simulink model "Clutchless_P2_Parallel_ETE"  (R2017b)
settings: Solver=FixedStepAuto  StartTime=0.0  StopTime=length(Speed)  FixedStep=0.01  MaxStep=0.01  RelTol=1e-3  EnableMultiTasking=on
PostLoadFcn:
  | , if any(exist('dsrtsu_mdlpostloadfcn', 'file') == [2, 3, 6]), try dsrtsu_mdlpostloadfcn('Execute', bdroot); catch fprintf('Error in PostLoadFcn (dsrtsu_mdlpostloadfcn) for model "%s":\n %s\n', bdroot, lasterr); end, end,
undefined symbols (not defined in the file): ABSEnable, Actuators, air, APP1_OOR, APP2_OOR, APP_Mismatch, Brk_Flt, cal, ClutchEngag, Clutchless_HSC_ETE, CS_On_Control, Driver, eng, Engine, EngOverTemp, ENGTRQ_MSMCH_Degraded_CP, ENGTRQ_MSMCH_ErrCritical_CP, ENGTRQ_MSMCH_LimpHome_CP, EngTrqMismatch, env, ess, ESSOverTemp, gb, KeyPos_Flt, KeyPosition, lib_Actuators, lib_Clutchless_HSC_ETE, lib_Driver, lib_EMachine_2017a, lib_Sensors_2017a, LossCAN, Machine, max_vehicle_rad_air_flow, MCUOverTemp, mot, MotDirMismatch, MotOverTemp, MotTrqMismatch, mph2ms, PRNDL_Flt, RegenBrkDisable, RegenFault, Sensors, ShiftLeverPosition, Speed, SW_CS_ON, SW_Engine_ON, t_amb, time, tloop
libraries: simulink x97, Pneumatic_lib x11, nesl_utility x9, EC2_libraries x7, powerlib_meascontrol x2, CalculationGallon x1, lib_Chassis x1, lib_DCDC x1, lib_Differential x1, lib_HVESS x1, fl_lib x1, lib_OBC x1
(part 8 of 9)

== system Clutchless_P2_Parallel_ETE/Clutchless_HSC_ETE/HSC/Camaro Fault Detection/Signal Diagnostic/Driver Signal Diagnostic/BrakeFailureDetection ==
  BPP : Inport
  VehSpeed : Inport  Port=2
  Trigger : TriggerPort  VariantControl=Variant  PortDimensions=1
  Chart : Stateflow chart  Commented=on  TreatAsAtomicUnit=on
  Compare To Constant : simulink/Logic and Bit Operations/Compare To Constant  relop=>  const=0  OutDataTypeStr=boolean
  Compare To Constant1 : simulink/Logic and Bit Operations/Compare To Constant  relop=>  const=0.5  OutDataTypeStr=boolean
  Detect Change : simulink/Logic and Bit Operations/Detect Change  vinit=0  InputProcessing=Inherited  OutDataTypeStr=boolean
  Detect Increase : simulink/Logic and Bit Operations/Detect Increase  vinit=0.0  InputProcessing=Inherited  OutDataTypeStr=boolean
  Logical Operator : Logic  Operator=NOT  AllPortsSameDT=off  OutDataTypeStr=boolean
  Logical Operator1 : Logic  AllPortsSameDT=off  OutDataTypeStr=boolean
  Logical Operator2 : Logic  Operator=OR  AllPortsSameDT=off  OutDataTypeStr=boolean
  Logical Operator3 : Logic  AllPortsSameDT=off  OutDataTypeStr=boolean
  Unit Delay : UnitDelay  SampleTime=-1
  Unit Delay1 : UnitDelay  SampleTime=-1
  DecelFail : Outport
  wires:
  VehSpeed/1 -> Unit Delay1/1, Detect Change/1, Detect Increase/1
  Detect Change/1 -> Logical Operator/1
  Compare To Constant/1 -> Logical Operator1/1
  Compare To Constant1/1 -> Logical Operator1/2
  BPP/1 -> Unit Delay/1
  Logical Operator1/1 -> Logical Operator3/1
  Detect Increase/1 -> Logical Operator2/1  "Increase"
  Logical Operator/1 -> Logical Operator2/2  "Unchange"
  Unit Delay/1 -> Compare To Constant/1
  Unit Delay1/1 -> Compare To Constant1/1
  Logical Operator2/1 -> Logical Operator3/2
  Logical Operator3/1 -> DecelFail/1

== system Clutchless_P2_Parallel_ETE/Clutchless_HSC_ETE/HSC/Camaro Fault Detection/Signal Diagnostic/Driver Signal Diagnostic/Latch ==
  In1 : Inport
  In2 : Inport  Port=2
  Memory : Memory
  NOT : Logic  Operator=NOT  OutDataTypeStr=boolean
  OR : Logic  OutDataTypeStr=boolean
  OR1 : Logic  Operator=OR  OutDataTypeStr=boolean
  Drv_APP_Agree : Outport
  wires:
  In1/1 -> OR1/1
  OR/1 -> OR1/2
  OR1/1 -> Drv_APP_Agree/1, Memory/1
  NOT/1 -> OR/1
  Memory/1 -> OR/2
  In2/1 -> NOT/1

== system Clutchless_P2_Parallel_ETE/Clutchless_HSC_ETE/HSC/Camaro Fault Detection/Signal Diagnostic/Driver Signal Diagnostic/Latch1 ==
  In1 : Inport
  In2 : Inport  Port=2
  Memory : Memory
  NOT : Logic  Operator=NOT  OutDataTypeStr=boolean
  OR : Logic  OutDataTypeStr=boolean
  OR1 : Logic  Operator=OR  OutDataTypeStr=boolean
  Out1 : Outport
  wires:
  In2/1 -> NOT/1
  Memory/1 -> OR/2
  NOT/1 -> OR/1
  OR1/1 -> Memory/1, Out1/1
  OR/1 -> OR1/2
  In1/1 -> OR1/1

== system Clutchless_P2_Parallel_ETE/Clutchless_HSC_ETE/HSC/Camaro Fault Detection/Signal Diagnostic/ESS Signal Diagnostic/Contactors status check ==
  note: Note: Contactors don't close when commanded
  In1 : Inport
  In2 : Inport  Port=2
  In3 : Inport  Port=3
  " " : simulink/Logic and Bit Operations/Compare To Constant  relop=>  const=0.5  OutDataTypeStr=boolean
  Abs : Abs
  Logical Operator : Logic  Operator=OR  AllPortsSameDT=off  OutDataTypeStr=boolean
  Sum : Sum  Inputs=+-
  Out1 : Outport
  wires:
  " "/1 -> Logical Operator/1  "BMS_contactorsFailed_SigValid"
  In3/1 -> Logical Operator/2
  In2/1 -> Sum/2
  Abs/1 -> " "/1
  Sum/1 -> Abs/1
  Logical Operator/1 -> Out1/1  "BMS_contactorsFailed_Detected"
  In1/1 -> Sum/1

== system Clutchless_P2_Parallel_ETE/Clutchless_HSC_ETE/HSC/Camaro Fault Detection/Signal Diagnostic/ESS Signal Diagnostic/ESS SOC Validity Check ==
  In1 : Inport
  Constant1 : Constant
  essSOCValidity_Check : Subsystem
  essSOC_0_1Range : Stateflow chart  TreatAsAtomicUnit=on
  Out1 : Outport
  Out2 : Outport  Port=2
  wires:
  essSOCValidity_Check/1(Out1) -> Out1/1  "BMS_essSOC_0_1_SigValid"
  In1/1 -> essSOC_0_1Range/2(signalValue)
  Constant1/1 -> essSOC_0_1Range/1(clearFaults)
  essSOC_0_1Range/1(essSOCRange) -> Out2/1, essSOCValidity_Check/1(In1)

== system Clutchless_P2_Parallel_ETE/Clutchless_HSC_ETE/HSC/Camaro Fault Detection/Signal Diagnostic/ESS Signal Diagnostic/ESS Temp Validity Check ==
  In1 : Inport
  Constant : Constant
  essTsignalRange : Stateflow chart  TreatAsAtomicUnit=on
  essTsignalValidity_Check : Subsystem
  Out1 : Outport
  Out2 : Outport  Port=2
  wires:
  Constant/1 -> essTsignalRange/1(clearFaults)
  essTsignalValidity_Check/1(Out1) -> Out1/1  "BMS_essTemp_[degC]_SigValid"
  essTsignalRange/1(essTempRange) -> Out2/1, essTsignalValidity_Check/1(In1)  "essTempRange[0_4]"
  In1/1 -> essTsignalRange/2(signalValue)

== system Clutchless_P2_Parallel_ETE/Clutchless_HSC_ETE/HSC/Camaro Fault Detection/Signal Diagnostic/ESS Signal Diagnostic/Max charging voltage fault detect ==
  note: Note: When the ESS receives the energy from grid or regenerative braking,
      | the charging voltage to the inverter can not be bigger than 419V, otherwise the MCU will set to fault
  In1 : Inport
  " " : simulink/Logic and Bit Operations/Compare To Constant  relop=>  const=419  OutDataTypeStr=boolean
  Abs : Abs
  Compare To Zero : simulink/Logic and Bit Operations/Compare To Zero  relop=<  OutDataTypeStr=boolean
  Logical Operator : Logic  AllPortsSameDT=off  OutDataTypeStr=boolean
  Out1 : Outport
  wires:
  Compare To Zero/1 -> Logical Operator/2
  In1/1 -> Abs/1, Compare To Zero/1
  " "/1 -> Logical Operator/1
  Logical Operator/1 -> Out1/1
  Abs/1 -> " "/1

== system Clutchless_P2_Parallel_ETE/Clutchless_HSC_ETE/HSC/Camaro Fault Detection/Signal Diagnostic/ESS Signal Diagnostic/Rolling Alive Counter Detection ==
  In1 : Inport
  Chart : Stateflow chart  TreatAsAtomicUnit=on
  Constant : Constant  Value=0.01
  Constant1 : Constant  Value=0.01
  Detect Change : simulink/Logic and Bit Operations/Detect Change  vinit=1  InputProcessing=Inherited  OutDataTypeStr=boolean
  Out1 : Outport
  wires:
  Constant/1 -> Chart/2(CycleTime)
  Chart/1(flag) -> Out1/1
  Detect Change/1 -> Chart/1(PulseDetect)
  In1/1 -> Detect Change/1
  Constant1/1 -> Chart/3(tloop)

== system Clutchless_P2_Parallel_ETE/Clutchless_HSC_ETE/HSC/Camaro Fault Detection/Signal Diagnostic/ESS Signal Diagnostic/Validity Check ==
  In1 : Inport
  " Normal Operation" : simulink/Logic and Bit Operations/Compare To Constant  relop===  const=1  OutDataTypeStr=boolean
  Below Normal Operation : simulink/Logic and Bit Operations/Compare To Constant  relop===  const=0  OutDataTypeStr=boolean
  Logical Operator : Logic  Operator=OR  AllPortsSameDT=off  OutDataTypeStr=boolean
  Out1 : Outport
  wires:
  Logical Operator/1 -> Out1/1  "BMSgdf_SigValid"
  " Normal Operation"/1 -> Logical Operator/2
  Below Normal Operation/1 -> Logical Operator/1
  In1/1 -> " Normal Operation"/1, Below Normal Operation/1

== system Clutchless_P2_Parallel_ETE/Clutchless_HSC_ETE/HSC/Camaro Fault Detection/Signal Diagnostic/Engine Signal Diagnostic/EngTempValidity_Check ==
  In1 : Inport
  Above Normal Operation : simulink/Logic and Bit Operations/Compare To Constant  relop===  const=3  OutDataTypeStr=boolean
  Logical Operator1 : Logic  Operator=NOT  AllPortsSameDT=off  OutDataTypeStr=boolean
  Out1 : Outport
  wires:
  In1/1 -> Above Normal Operation/1
  Above Normal Operation/1 -> Logical Operator1/1
  Logical Operator1/1 -> Out1/1

== system Clutchless_P2_Parallel_ETE/Clutchless_HSC_ETE/HSC/Camaro Fault Detection/Signal Diagnostic/Engine Signal Diagnostic/Rolling Alive Counter Detection1 ==
  In1 : Inport
  Chart : Stateflow chart  TreatAsAtomicUnit=on
  Constant : Constant  Value=0.01
  Detect Change : simulink/Logic and Bit Operations/Detect Change  vinit=1  InputProcessing=Inherited  OutDataTypeStr=boolean
  Out1 : Outport
  wires:
  In1/1 -> Detect Change/1
  Detect Change/1 -> Chart/1(PulseDetect)
  Chart/1(flag) -> Out1/1
  Constant/1 -> Chart/2(CycleTime)

== system Clutchless_P2_Parallel_ETE/Clutchless_HSC_ETE/HSC/Camaro Fault Detection/Signal Diagnostic/Transmission Signal Diagnostic/Rolling Alive Counter Detection ==
  In1 : Inport
  Chart : Stateflow chart  TreatAsAtomicUnit=on
  Constant : Constant  Value=0.01
  Detect Change : simulink/Logic and Bit Operations/Detect Change  vinit=1  InputProcessing=Inherited  OutDataTypeStr=boolean
  Out1 : Outport
  wires:
  In1/1 -> Detect Change/1
  Detect Change/1 -> Chart/1(PulseDetect)
  Chart/1(flag) -> Out1/1
  Constant/1 -> Chart/2(CycleTime)

== system Clutchless_P2_Parallel_ETE/Clutchless_HSC_ETE/HSC/Camaro Fault Detection/Signal Diagnostic/Transmission Signal Diagnostic/Vehicle Direction Fault Detection ==
  LvrPosTrnsShft : Inport
  Speed : Inport  Port=2
  Compare To Constant : simulink/Logic and Bit Operations/Compare To Constant  relop===  const=4  OutDataTypeStr=boolean
  Compare To Constant1 : simulink/Logic and Bit Operations/Compare To Constant  relop=<  const=0  OutDataTypeStr=boolean
  Compare To Constant2 : simulink/Logic and Bit Operations/Compare To Constant  relop===  const=2  OutDataTypeStr=boolean
  Compare To Constant3 : simulink/Logic and Bit Operations/Compare To Constant  relop=>  const=0  OutDataTypeStr=boolean
  Logical Operator : Logic  AllPortsSameDT=off  OutDataTypeStr=boolean
  Logical Operator1 : Logic  AllPortsSameDT=off  OutDataTypeStr=boolean
  Logical Operator2 : Logic  Operator=OR  AllPortsSameDT=off  OutDataTypeStr=boolean
  Out1 : Outport
  wires:
  LvrPosTrnsShft/1 -> Compare To Constant2/1, Compare To Constant/1
  Speed/1 -> Compare To Constant3/1, Compare To Constant1/1
  Compare To Constant1/1 -> Logical Operator/2
  Compare To Constant/1 -> Logical Operator/1
  Compare To Constant2/1 -> Logical Operator1/1
  Compare To Constant3/1 -> Logical Operator1/2
  Logical Operator1/1 -> Logical Operator2/1
  Logical Operator/1 -> Logical Operator2/2
  Logical Operator2/1 -> Out1/1

== system Clutchless_P2_Parallel_ETE/Clutchless_HSC_ETE/HSC/Driver_Requests/APP_BPP to DrvIntndAxlTrq2/Post Driver Intnded Axle Torque/Brake Command ==
  APP : Inport
  BPP : Inport  Port=2
  VehicleSpeed : Inport  Port=3
  1-D Lookup Table : Lookup_n-D  NumberOfTableDimensions=1  BreakpointsForDimension1=cal.Regen.BrakeAxleTrq.idx1_BrkPdlPos  Table=cal.Regen.BrakeAxleTrq.map  InternalRulePriority=Speed  RndMeth=Simplest  InputSameDT=on
  Compare To Constant : simulink/Logic and Bit Operations/Compare To Constant  relop=>=  const=cal.Regen.EnableSpeed  OutDataTypeStr=boolean
  Compare To Constant4 : simulink/Logic and Bit Operations/Compare To Constant  relop=<=  const=cal.Regen.EnableAPP  OutDataTypeStr=boolean
  Compare To Constant5 : simulink/Logic and Bit Operations/Compare To Constant  relop=>=  const=cal.Regen.DisableAPP  OutDataTypeStr=boolean
  Constant5 : Constant  Value=0
  Latch : Subsystem
  RegenCal : Gain  Gain=1.3
  Switch : Switch  Criteria=u2 > Threshold  Threshold=1
  Terminator : Terminator
  BrkAxlTrq : Outport
  wires:
  RegenCal/1 -> Switch/1
  Latch/1(Out1) -> Terminator/1
  Compare To Constant4/1 -> Latch/1(Input)
  Compare To Constant5/1 -> Latch/2(Reset)
  Constant5/1 -> Switch/3
  Compare To Constant/1 -> Switch/2
  BPP/1 -> 1-D Lookup Table/1
  APP/1 -> Compare To Constant4/1, Compare To Constant5/1
  Switch/1 -> BrkAxlTrq/1
  1-D Lookup Table/1 -> RegenCal/1
  VehicleSpeed/1 -> Compare To Constant/1

== system Clutchless_P2_Parallel_ETE/Clutchless_HSC_ETE/HSC/Driver_Requests/APP_BPP to DrvIntndAxlTrq2/Post Driver Intnded Axle Torque/Driver Intended Axle Torque ==
  note: //*mode==1 (CD Mode)
      | mode==2 (CS Mode - Engine Drive)
      | mode==3 (CS Mode-Motor Drive) pass MotTrq
      | mode==4 (Sports Mode) pass Mot Trq+Eng Trq
      | mode==5 (Engine Charging mode)
      | mode==66 (Engine Only mode)*//
  note: In Engine Only mode, ETAS is only as a gateway to broadcast CAN messages
  APP : Inport
  Mode : Inport  Port=2
  TransGearRatio : Inport  Port=3
  Compare To Constant1 : simulink/Logic and Bit Operations/Compare To Constant  relop===  const=2  OutDataTypeStr=boolean
  Compare To Constant2 : simulink/Logic and Bit Operations/Compare To Constant  relop===  const=4  OutDataTypeStr=boolean
  Compare To Constant3 : simulink/Logic and Bit Operations/Compare To Constant  relop===  const=5  OutDataTypeStr=boolean
  Compare To Constant4 : simulink/Logic and Bit Operations/Compare To Constant  relop===  const=1  OutDataTypeStr=boolean
  Compare To Constant5 : simulink/Logic and Bit Operations/Compare To Constant  relop===  const=3  OutDataTypeStr=boolean
  Compare To Constant6 : simulink/Logic and Bit Operations/Compare To Constant  relop===  const=66  OutDataTypeStr=boolean
  Constant : Constant  Value=eng.plant.trq_max_hot_point  VectorParams1D=off
  Constant1 : Constant  Value=fd.plant.init.ratio
  Constant2 : Constant  Value=mot.plant.init.motor.trq_max.points.trq  VectorParams1D=off
  Constant3 : Constant  Value=mot.plant.init.motor.trq_max.points.trq  VectorParams1D=off
  Constant4 : Constant  Value=eng.plant.trq_max_hot_point  VectorParams1D=off
  Gain1 : Gain  Gain=1/100
  Gain2 : Gain  Gain=1/100
  Gain3 : Gain  Gain=1/100
  Logical Operator : Logic  Operator=OR  Inputs=4  AllPortsSameDT=off  OutDataTypeStr=boolean
  Logical Operator1 : Logic  Operator=OR  AllPortsSameDT=off  OutDataTypeStr=boolean
  Memory : Memory
  Product : Product  RndMeth=Zero
  Product1 : Product  RndMeth=Zero
  Product2 : Product  Inputs=3  RndMeth=Zero
  Product3 : Product  RndMeth=Zero
  Ratio Filter : Subsystem
  Sum1 : Sum
  Switch1 : Switch  Threshold=1
  Switch3 : Switch  Threshold=1
  Out1 : Outport
  wires:
  Compare To Constant5/1 -> Logical Operator/4
  Compare To Constant4/1 -> Logical Operator/3
  Compare To Constant6/1 -> Logical Operator1/2
  Logical Operator1/1 -> Switch1/2
  Gain3/1 -> Product3/1
  Constant4/1 -> Product3/2
  APP/1 -> Gain1/1, Gain3/1, Gain2/1
  Memory/1 -> Compare To Constant5/1, Compare To Constant4/1, Compare To Constant1/1, Compare To Constant6/1, Compare To Constant3/1, Compare To Constant2/1
  Compare To Constant3/1 -> Logical Operator1/1
  Switch1/1 -> Product2/1
  Product3/1 -> Switch1/1, [IntdAxleTrq_eng]
  Logical Operator/1 -> Switch3/2
  Switch3/1 -> Switch1/3  "DrvIntndAxlTrq"
  Constant/1 -> Sum1/2
  Compare To Constant2/1 -> Logical Operator/2
  Sum1/1 -> Product/1
  Compare To Constant1/1 -> Logical Operator/1
  Constant3/1 -> Sum1/1
  Gain1/1 -> Product/2
  Product2/1 -> Out1/1  "DrvIntndAxlTrq"
  TransGearRatio/1 -> Ratio Filter/1(Ratio)
  Product1/1 -> Switch3/3
  Constant1/1 -> Product2/3  "ratio"
  Mode/1 -> Memory/1
  Product/1 -> Switch3/1
  Gain2/1 -> Product1/2
  Ratio Filter/1(Filtered_Ratio) -> Product2/2
  Constant2/1 -> Product1/1

== system Clutchless_P2_Parallel_ETE/Clutchless_HSC_ETE/HSC/Powertrain Manager/HV Manager1/BMS_Manager/Fault Latch ==
  IsoFault : Inport
  Off Delay : powerlib_meascontrol/Logic/On Delay  DelayType=Off delay  delay=3  ic=0  Ts=0
      settings: SourceProductName=Simscape Power Systems
  IsoFaultLatched : Outport
  wires:
  Off Delay/1 -> IsoFaultLatched/1
  IsoFault/1 -> Off Delay/1

== system Clutchless_P2_Parallel_ETE/Clutchless_HSC_ETE/HSC/Powertrain Manager/HV Manager1/BMS_Manager/ISO_Hybrid_01_Req ==
  In1 : Inport
  Bus Creator : BusCreator  Inputs=9
  ISO_Hybrid_01_Req_Data_byte_0 : Constant  Value=3
  ISO_Hybrid_01_Req_Data_byte_1 : Constant  Value=34
  ISO_Hybrid_01_Req_Data_byte_2 : Constant  Value=30
  ISO_Hybrid_01_Req_Data_byte_3 : Constant  Value=25
  ISO_Hybrid_01_Req_Data_byte_{4..7} (4 alike) : Constant  Value=0
  ISO_Hybrid_01_Req_Data_byte_8 : Constant  Value=23
  ISO_Request : DiscretePulseGenerator  PulseType=Time based  Period=0.5  PulseWidth=50  SampleTime=-1
  Switch{,1..8} (9 alike) : Switch  Criteria=u2 > Threshold
  Out1 : Outport
  wires:
  ISO_Request/1 -> Switch/2  "<ISO_Hybrid_01_Req_Data_byte_3>"
  ISO_Hybrid_01_Req_Data_byte_7/1 -> Switch8/1
  ISO_Hybrid_01_Req_Data_byte_6/1 -> Switch7/1
  ISO_Hybrid_01_Req_Data_byte_5/1 -> Switch6/1
  ISO_Hybrid_01_Req_Data_byte_4/1 -> Switch5/1
  Switch/1 -> Switch4/1  "ISO_Hybrid_01_Req_Data_byte_3"
  ISO_Hybrid_01_Req_Data_byte_2/1 -> Switch3/1
  ISO_Hybrid_01_Req_Data_byte_1/1 -> Switch2/1
  In1/1 -> Switch1/2, Switch1/3, Switch2/3, Switch3/2, Switch4/2, Switch5/2, Switch6/2, Switch8/3, Bus Creator/9, Switch8/2, Switch7/3, Switch7/2, Switch6/3, Switch5/3, Switch4/3, Switch3/3, Switch2/2
  ISO_Hybrid_01_Req_Data_byte_0/1 -> Switch1/1
  Switch4/1 -> Bus Creator/4  "ISO_Hybrid_01_Req_Data_byte_3"
  Switch8/1 -> Bus Creator/8  "ISO_Hybrid_01_Req_Data_byte_7"
  Switch2/1 -> Bus Creator/2  "ISO_Hybrid_01_Req_Data_byte_1"
  Switch7/1 -> Bus Creator/7  "ISO_Hybrid_01_Req_Data_byte_6"
  Switch1/1 -> Bus Creator/1  "ISO_Hybrid_01_Req_Data_byte_0"
  ISO_Hybrid_01_Req_Data_byte_3/1 -> Switch/1
  Switch3/1 -> Bus Creator/3  "ISO_Hybrid_01_Req_Data_byte_2"
  Switch5/1 -> Bus Creator/5  "ISO_Hybrid_01_Req_Data_byte_4"
  ISO_Hybrid_01_Req_Data_byte_8/1 -> Switch/3
  Switch6/1 -> Bus Creator/6  "ISO_Hybrid_01_Req_Data_byte_5"
  Bus Creator/1 -> Out1/1  "ISO_Hybrid_01_Req"

== system Clutchless_P2_Parallel_ETE/Clutchless_HSC_ETE/HSC/Powertrain Manager/HV Manager1/BMS_Manager/Isolation Fault Calculation ==
  note: This block  allows to know which HV main
      | is having issues. HV POS 25, HV NEG 23.
  Sensors1 : Inport
  Bus Selector5 : BusSelector  OutputSignals=from_CAN.fromEBCAN.from_BMSAntrieb.ISO_Hybrid_01_Resp_Data.ISO_Hybrid_01_Resp_Data_byte_3,from_CAN.fromEBCAN.from_BMSAntrieb.ISO_Hybrid_01_Resp_Data.ISO_Hybrid_01_Resp_Data_byte_4,from_CAN.fromEBCAN.from_BMSAntrieb.ISO_Hybrid_01_Resp_Data.ISO_Hybrid_01_Resp_Data_byte_5
  Compare To Constant : simulink/Logic and Bit Operations/Compare To Constant  relop===  const=23  OutDataTypeStr=boolean
  Compare To Constant1 : simulink/Logic and Bit Operations/Compare To Constant  relop===  const=25  OutDataTypeStr=boolean
  HVnegativeISO : Constant  Value=0
  HVpositiveISO : Constant
  Logical Operator : Logic  Operator=OR  AllPortsSameDT=off  OutDataTypeStr=boolean
  POS or NEG HV MAIN : Switch  Criteria=u2 > Threshold  Threshold=24
  Resistance_Measurement : Subsystem
  Terminator8 : Terminator
  IsoFault : Outport
  wires:
  Logical Operator/1 -> Resistance_Measurement/Enable
  Compare To Constant/1 -> Logical Operator/2
  Compare To Constant1/1 -> Logical Operator/1
  HVnegativeISO/1 -> POS or NEG HV MAIN/3
  Bus Selector5/1 -> Compare To Constant/1, Compare To Constant1/1, POS or NEG HV MAIN/2  "<ISO_Hybrid_01_Resp_Data_byte_3>"
  HVpositiveISO/1 -> POS or NEG HV MAIN/1
  Sensors1/1 -> Bus Selector5/1
  Bus Selector5/3 -> Resistance_Measurement/2(In2)  "<ISO_Hybrid_01_Resp_Data_byte_5>"
  Bus Selector5/2 -> Resistance_Measurement/1(In1)  "<ISO_Hybrid_01_Resp_Data_byte_4>"
  POS or NEG HV MAIN/1 -> Terminator8/1
  Resistance_Measurement/1(IsoFault) -> IsoFault/1

== system Clutchless_P2_Parallel_ETE/Clutchless_HSC_ETE/HSC/Powertrain Manager/HV Manager1/DCDC Manager/Contactors status check ==
  note: Note: Contactors don't close when commanded
  In1 : Inport
  " " : simulink/Logic and Bit Operations/Compare To Constant  relop=>  const=5  OutDataTypeStr=boolean
  Abs : Abs
  Bus Selector1 : BusSelector  OutputSignals=from_CAN.fromHV_CAN.from_BMSHybrid.BMS_HYB_02.BMS_IstSpannung,from_CAN.fromHV_CAN.from_BMSHybrid.BMS_Spannung_ZwKr,from_CAN.fromHV_CAN.from_BMSHybrid.BMS_HYB_02.BMS_Fehler_Pilot
  Logical Operator : Logic  Operator=OR  AllPortsSameDT=off  OutDataTypeStr=boolean
  Sum : Sum  Inputs=+-
  Out1 : Outport
  wires:
  Bus Selector1/2 -> Sum/2  "<BMS_Spannung_ZwKr>"
  Bus Selector1/3 -> Logical Operator/2  "<BMS_Fehler_Pilot>"
  In1/1 -> Bus Selector1/1
  " "/1 -> Logical Operator/1  "BMS_contactorsFailed_SigValid"
  Abs/1 -> " "/1
  Sum/1 -> Abs/1
  Logical Operator/1 -> Out1/1  "BMS_contactorsFailed_Detected"
  Bus Selector1/1 -> Sum/1  "<BMS_IstSpannung>"

== system Clutchless_P2_Parallel_ETE/Clutchless_HSC_ETE/HSC/Powertrain Manager/HV Manager1/DCDC Manager/Override_Current ==
  In1 : Inport
  CurrentHVOvrrdSW : Constant  Value=0
  CurrentHVOvrrdVAL : Constant  Value=20
  Switch : Switch  Criteria=u2 > Threshold
  Out1 : Outport
  wires:
  CurrentHVOvrrdVAL/1 -> Switch/1
  CurrentHVOvrrdSW/1 -> Switch/2
  In1/1 -> Switch/3
  Switch/1 -> Out1/1  "DC_mode"

== system Clutchless_P2_Parallel_ETE/Clutchless_HSC_ETE/HSC/Powertrain Manager/HV Manager1/DCDC Manager/Override_CurrentLV ==
  In1 : Inport
  CurrentLVOvrrdSW : Constant  Value=0
  CurrentLVOvrrdVAL : Constant  Value=173
  Switch : Switch  Criteria=u2 > Threshold
  Out1 : Outport
  wires:
  CurrentLVOvrrdVAL/1 -> Switch/1
  CurrentLVOvrrdSW/1 -> Switch/2
  In1/1 -> Switch/3
  Switch/1 -> Out1/1  "DC_mode"

== system Clutchless_P2_Parallel_ETE/Clutchless_HSC_ETE/HSC/Powertrain Manager/HV Manager1/DCDC Manager/Override_Voltage ==
  In1 : Inport
  Switch : Switch  Criteria=u2 > Threshold
  VoltageHVOvrrdSW : Constant  Value=0
  voltageHVOvrrdVal : Constant  Value=0
  Out1 : Outport
  wires:
  Switch/1 -> Out1/1  "DC_mode"
  In1/1 -> Switch/3
  VoltageHVOvrrdSW/1 -> Switch/2
  voltageHVOvrrdVal/1 -> Switch/1

== system Clutchless_P2_Parallel_ETE/Clutchless_HSC_ETE/HSC/Powertrain Manager/HV Manager1/DCDC Manager/Override_VoltageLV ==
  In1 : Inport
  Switch : Switch  Criteria=u2 > Threshold
  VoltageLVOvrrdSW : Constant  Value=0
  VoltageLVOvrrdVAL : Constant  Value=14
  Out1 : Outport
  wires:
  Switch/1 -> Out1/1  "DC_mode"
  In1/1 -> Switch/3
  VoltageLVOvrrdSW/1 -> Switch/2
  VoltageLVOvrrdVAL/1 -> Switch/1

== system Clutchless_P2_Parallel_ETE/Clutchless_HSC_ETE/HSC/Powertrain Manager/HV Manager1/DCDC Manager/Override_mode ==
  In1 : Inport
  DCDCOVrrdSwitch : Constant  Value=0
  DCDCOVrrdVal : Constant  Value=0
  Switch : Switch  Criteria=u2 > Threshold
  Out1 : Outport
  wires:
  DCDCOVrrdVal/1 -> Switch/1
  DCDCOVrrdSwitch/1 -> Switch/2
  In1/1 -> Switch/3
  Switch/1 -> Out1/1  "DC_mode"

== system Clutchless_P2_Parallel_ETE/Clutchless_HSC_ETE/HSC/Powertrain Manager/Torque Distribution/AxlTrq_to_EngTrq/Ratio Filter ==
  Ratio : Inport
  Abs : Abs
  Compare To Zero : simulink/Logic and Bit Operations/Compare To Zero  relop===  OutDataTypeStr=boolean
  Constant : Constant  Value=cal.Time.TrnsOvrllEstTrqRatioSwitch
  Mature_Delay : EC2_libraries/Mature_Delay
  Memory1 : Memory  InitialCondition=1
  Switch1 : Switch  Threshold=1
  Switch2 : Switch  Threshold=1
  Filtered_Ratio : Outport
  wires:
  Switch2/1 -> Memory1/1, Filtered_Ratio/1  "gear_ratio"
  Memory1/1 -> Switch1/3
  Mature_Delay/1 -> Switch1/2
  Constant/1 -> Mature_Delay/2
  Switch1/1 -> Switch2/1
  Abs/1 -> Switch2/3, Switch1/1
  Compare To Zero/1 -> Switch2/2, Mature_Delay/1
  Ratio/1 -> Abs/1, Compare To Zero/1

== system Clutchless_P2_Parallel_ETE/Clutchless_HSC_ETE/HSC/Powertrain Manager/Torque Distribution/AxlTrq_to_MotTrq/AxlTrq_to_MtrTrq2 ==
  note: //From motor axle torque to motor torque//
  In1 : Inport
  Compare To Constant : simulink/Logic and Bit Operations/Compare To Constant  relop===  const=0  OutDataTypeStr=boolean
  Constant1 : Constant  Value=max(gb.plant.init.ratio.map)
  Constant5 : Constant  Value=fd.plant.init.ratio
  Divide : Product  Inputs=*//
  Rate Limiter : RateLimiter  RisingSlewLimit=mcu.plant.init.trq_uprate  FallingSlewLimit=mcu.plant.init.trq_derate
  Ratio Filter : Subsystem
  Switch : Switch  Criteria=u2 > Threshold
  MtrTrqCmd : Outport
  wires:
  Ratio Filter/1(Filtered_Ratio) -> Compare To Constant/1, Switch/3
  Switch/1 -> Divide/3
  Rate Limiter/1 -> MtrTrqCmd/1
  Constant1/1 -> Switch/1
  Compare To Constant/1 -> Switch/2
  [TransRatio] -> Ratio Filter/1(Ratio)
  Divide/1 -> Rate Limiter/1
  Constant5/1 -> Divide/2
  In1/1 -> Divide/1

== system Clutchless_P2_Parallel_ETE/Clutchless_HSC_ETE/HSC/Powertrain Manager/Torque Distribution/AxlTrq_to_MotTrq/electric machine filter ==
  trq : Inport
  Interval Test : simulink/Logic and Bit Operations/Interval Test  IntervalClosedRight=on  uplimit=0.02  IntervalClosedLeft=on  lowlimit=-0.02  OutDataTypeStr=boolean
  Switch : Switch  Threshold=0.5
  electric machine time response : TransferFcn  Denominator=[mot.plant.init.time_response 1]
  filtered : Outport
  wires:
  Switch/1 -> filtered/1
  trq/1 -> Switch/1, electric machine time response/1, Interval Test/1
  Interval Test/1 -> Switch/2
  electric machine time response/1 -> Switch/3

== system Clutchless_P2_Parallel_ETE/Clutchless_HSC_ETE/HSC/Powertrain Manager/Torque Distribution/Supervisory  Control  Logic/VehReady.Eng_Charging_Stat.EngTrqCalc/Multiply by Zero Fix ==
  In1 : Inport
  Compare To Constant : simulink/Logic and Bit Operations/Compare To Constant  relop===  const=0  OutDataTypeStr=boolean
  Constant1 : Constant  Value=max(gb.plant.init.ratio.map)
  Ratio Filter : Subsystem
  Switch : Switch  Criteria=u2 > Threshold
  Out1 : Outport
  wires:
  In1/1 -> Ratio Filter/1(Ratio)
  Constant1/1 -> Switch/1
  Switch/1 -> Out1/1
  Compare To Constant/1 -> Switch/2
  Ratio Filter/1(Filtered_Ratio) -> Compare To Constant/1, Switch/3

== system Clutchless_P2_Parallel_ETE/Camaro Plant Model/E-Machine/IMG Plant/Electric Machine/Thermal1/MotInv_loop/MCUOverTemp Fault ==
  In1 : Inport
  Gain : Gain  Gain=3
  Switch : Switch  Threshold=1
  Out1 : Outport
  wires:
  Switch/1 -> Out1/1
  Gain/1 -> Switch/1
  [MCUOverTemp] -> Switch/2
  In1/1 -> Gain/1, Switch/3

== system Clutchless_P2_Parallel_ETE/Camaro Plant Model/E-Machine/IMG Plant/Electric Machine/Thermal1/MotInv_loop/MotorOverTempFault ==
  In1 : Inport
  Gain : Gain  Gain=2
  Memory : Memory
  Switch1 : Switch  Threshold=1
  Out1 : Outport
  wires:
  Switch1/1 -> Out1/1
  Gain/1 -> Switch1/1
  [MotOverTemp] -> Switch1/2
  In1/1 -> Switch1/3, Memory/1
  Memory/1 -> Gain/1

== system Clutchless_P2_Parallel_ETE/Camaro Plant Model/E-Machine/IMG Plant/Electric Machine/Thermal1/Motor Thermal/Lower Limit ==
  In1 : Inport
  Constant3 : Constant  Value=Lolimit
  MinMax : MinMax  Function=max  Inputs=2
  Out1 : Outport
  wires:
  MinMax/1 -> Out1/1
  Constant3/1 -> MinMax/2
  In1/1 -> MinMax/1

== system Clutchless_P2_Parallel_ETE/Camaro Plant Model/E-Machine/Soft MCU/Torque Calculation1/max torque /Heat index/Divide ==
  note: Take care of
      | division by 0
  numerator : Inport
  denominator : Inport  Port=2
  Fcn : Fcn  Expr=u[1] / ( u[2] + eps*(u[2]==0) )
  Mux : Mux  Inputs=2
  quotient : Outport
  wires:
  denominator/1 -> Mux/2
  Fcn/1 -> quotient/1
  numerator/1 -> Mux/1
  Mux/1 -> Fcn/1

== system Clutchless_P2_Parallel_ETE/Camaro Plant Model/E-Machine/Soft MCU/Torque Calculation2/max torque /Heat index/Divide ==
  note: Take care of
      | division by 0
  numerator : Inport
  denominator : Inport  Port=2
  Fcn : Fcn  Expr=u[1] / ( u[2] + eps*(u[2]==0) )
  Mux : Mux  Inputs=2
  quotient : Outport
  wires:
  denominator/1 -> Mux/2
  Fcn/1 -> quotient/1
  numerator/1 -> Mux/1
  Mux/1 -> Fcn/1

== system Clutchless_P2_Parallel_ETE/Clutchless_HSC_ETE/HSC/Camaro Fault Detection/Signal Diagnostic/ESS Signal Diagnostic/ESS SOC Validity Check/essSOCValidity_Check ==
  In1 : Inport
  Above Normal Operation : simulink/Logic and Bit Operations/Compare To Constant  relop===  const=3  OutDataTypeStr=boolean
  Below Normal Operation : simulink/Logic and Bit Operations/Compare To Constant  relop===  const=0  OutDataTypeStr=boolean
  Logical Operator : Logic  Operator=OR  AllPortsSameDT=off  OutDataTypeStr=boolean
  Logical Operator1 : Logic  Operator=NOT  AllPortsSameDT=off  OutDataTypeStr=boolean
  Out1 : Outport
  wires:
  Logical Operator1/1 -> Out1/1
  Above Normal Operation/1 -> Logical Operator/2
  Below Normal Operation/1 -> Logical Operator/1
  Logical Operator/1 -> Logical Operator1/1
  In1/1 -> Below Normal Operation/1, Above Normal Operation/1

== system Clutchless_P2_Parallel_ETE/Clutchless_HSC_ETE/HSC/Camaro Fault Detection/Signal Diagnostic/ESS Signal Diagnostic/ESS Temp Validity Check/essTsignalValidity_Check ==
  In1 : Inport
  Above Normal Operation : simulink/Logic and Bit Operations/Compare To Constant  relop===  const=4  OutDataTypeStr=boolean
  Below Normal Operation : simulink/Logic and Bit Operations/Compare To Constant  relop===  const=0  OutDataTypeStr=boolean
  Logical Operator : Logic  Operator=OR  AllPortsSameDT=off  OutDataTypeStr=boolean
  Logical Operator1 : Logic  Operator=NOT  AllPortsSameDT=off  OutDataTypeStr=boolean
  Out1 : Outport
  wires:
  In1/1 -> Above Normal Operation/1, Below Normal Operation/1
  Logical Operator/1 -> Logical Operator1/1
  Below Normal Operation/1 -> Logical Operator/1
  Above Normal Operation/1 -> Logical Operator/2
  Logical Operator1/1 -> Out1/1

== system Clutchless_P2_Parallel_ETE/Clutchless_HSC_ETE/HSC/Driver_Requests/APP_BPP to DrvIntndAxlTrq2/Post Driver Intnded Axle Torque/Brake Command/Latch ==
  Input : Inport
  Reset : Inport  Port=2
  Logical Operator1 : Logic  Operator=NOT  AllPortsSameDT=off  OutDataTypeStr=boolean
  Logical Operator2 : Logic  AllPortsSameDT=off  OutDataTypeStr=boolean
  Logical Operator3 : Logic  Operator=OR  AllPortsSameDT=off  OutDataTypeStr=boolean
  Memory1 : Memory
  Out1 : Outport
  wires:
  Input/1 -> Logical Operator3/1
  Logical Operator1/1 -> Logical Operator2/1
  Logical Operator3/1 -> Memory1/1, Out1/1
  Memory1/1 -> Logical Operator2/2
  Reset/1 -> Logical Operator1/1
  Logical Operator2/1 -> Logical Operator3/2

== system Clutchless_P2_Parallel_ETE/Clutchless_HSC_ETE/HSC/Driver_Requests/APP_BPP to DrvIntndAxlTrq2/Post Driver Intnded Axle Torque/Driver Intended Axle Torque/Ratio Filter ==
  Ratio : Inport
  Abs : Abs
  Compare To Zero : simulink/Logic and Bit Operations/Compare To Zero  relop===  OutDataTypeStr=boolean
  Constant : Constant  Value=cal.Time.TrnsOvrllEstTrqRatioSwitch
  Mature_Delay : EC2_libraries/Mature_Delay
  Memory1 : Memory  InitialCondition=1
  Switch1 : Switch  Threshold=1
  Switch2 : Switch  Threshold=1
  Filtered_Ratio : Outport
  wires:
  Switch2/1 -> Memory1/1, Filtered_Ratio/1  "gear_ratio"
  Memory1/1 -> Switch1/3
  Mature_Delay/1 -> Switch1/2
  Constant/1 -> Mature_Delay/2
  Switch1/1 -> Switch2/1
  Abs/1 -> Switch2/3, Switch1/1
  Compare To Zero/1 -> Switch2/2, Mature_Delay/1
  Ratio/1 -> Abs/1, Compare To Zero/1

== system Clutchless_P2_Parallel_ETE/Clutchless_HSC_ETE/HSC/Powertrain Manager/HV Manager1/BMS_Manager/Isolation Fault Calculation/Resistance_Measurement ==
  In1 : Inport
  In2 : Inport  Port=2
  Enable : EnablePort
  Add : Sum
  ISOfault : Constant
  ISOmultiplier : Constant  Value=256
  ISOnofault : Constant  Value=0
  Minimum Allowed Isolation Resistance : Switch  Criteria=u2 > Threshold  Threshold=500000
  Product : Product
  Product1 : Product
  Resistance Adjustment : Constant  Value=1000
  IsoFault : Outport
  wires:
  ISOmultiplier/1 -> Product/2
  In1/1 -> Product/1
  In2/1 -> Add/2
  Product/1 -> Add/1
  Add/1 -> Product1/1
  ISOfault/1 -> Minimum Allowed Isolation Resistance/3
  Product1/1 -> Minimum Allowed Isolation Resistance/2
  Resistance Adjustment/1 -> Product1/2
  ISOnofault/1 -> Minimum Allowed Isolation Resistance/1
  Minimum Allowed Isolation Resistance/1 -> IsoFault/1  "IsoFault"

== system Clutchless_P2_Parallel_ETE/Clutchless_HSC_ETE/HSC/Powertrain Manager/Torque Distribution/AxlTrq_to_MotTrq/AxlTrq_to_MtrTrq2/Ratio Filter ==
  Ratio : Inport
  Abs : Abs
  Compare To Zero : simulink/Logic and Bit Operations/Compare To Zero  relop===  OutDataTypeStr=boolean
  Constant : Constant  Value=cal.Time.TrnsOvrllEstTrqRatioSwitch
  Mature_Delay : EC2_libraries/Mature_Delay
  Memory1 : Memory  InitialCondition=1
  Switch1 : Switch  Threshold=1
  Switch2 : Switch  Threshold=1
  Filtered_Ratio : Outport
  wires:
  Switch2/1 -> Memory1/1, Filtered_Ratio/1  "gear_ratio"
  Memory1/1 -> Switch1/3
  Mature_Delay/1 -> Switch1/2
  Constant/1 -> Mature_Delay/2
  Switch1/1 -> Switch2/1
  Abs/1 -> Switch2/3, Switch1/1
  Compare To Zero/1 -> Switch2/2, Mature_Delay/1
  Ratio/1 -> Abs/1, Compare To Zero/1

== system Clutchless_P2_Parallel_ETE/Clutchless_HSC_ETE/HSC/Powertrain Manager/Torque Distribution/Supervisory  Control  Logic/VehReady.Eng_Charging_Stat.EngTrqCalc/Multiply by Zero Fix/Ratio Filter ==
  Ratio : Inport
  Abs : Abs
  Compare To Zero : simulink/Logic and Bit Operations/Compare To Zero  relop===  OutDataTypeStr=boolean
  Constant : Constant  Value=cal.Time.TrnsOvrllEstTrqRatioSwitch
  Mature_Delay : Subsystem  AncestorBlock=EC2_libraries/Mature_Delay
  Memory1 : Memory  InitialCondition=1  InheritSampleTime=on
  Switch1 : Switch  Threshold=1
  Switch2 : Switch  Threshold=1
  Filtered_Ratio : Outport
  wires:
  Switch2/1 -> Memory1/1, Filtered_Ratio/1  "gear_ratio"
  Memory1/1 -> Switch1/3
  Mature_Delay/1(Out) -> Switch1/2
  Constant/1 -> Mature_Delay/2(MatTime)
  Switch1/1 -> Switch2/1
  Abs/1 -> Switch2/3, Switch1/1
  Compare To Zero/1 -> Switch2/2, Mature_Delay/1(In)
  Ratio/1 -> Abs/1, Compare To Zero/1

== system Clutchless_P2_Parallel_ETE/Clutchless_HSC_ETE/HSC/Powertrain Manager/Torque Distribution/Supervisory  Control  Logic/VehReady.Eng_Charging_Stat.EngTrqCalc/Multiply by Zero Fix/Ratio Filter/Mature_Delay ==
  In : Inport
  MatTime : Inport  Port=2
  Gain : Gain  Gain=-1
  Lower Limit : EC2_libraries/Lower Limit  Lolimit=0.001
  Memory1 : Memory  InheritSampleTime=on
  Relational Operator1 : RelationalOperator  Operator=>  OutDataTypeStr=boolean  RndMeth=Nearest
  StepTm[sec] : Constant  Value=tloop
  Sum : Sum  Inputs=|++
  Switch1 : Switch  Threshold=1
  Out : Outport
  wires:
  In/1 -> Switch1/2
  Gain/1 -> Switch1/3
  Memory1/1 -> Sum/2, Gain/1
  Relational Operator1/1 -> Out/1
  MatTime/1 -> Relational Operator1/2
  StepTm[sec]/1 -> Switch1/1
  Switch1/1 -> Sum/1
  Sum/1 -> Memory1/1, Lower Limit/1
  Lower Limit/1 -> Relational Operator1/1

== matlab function Clutchless_P2_Parallel_ETE/Camaro Plant Model/E-Machine/Soft MCU/diff_INV_state ==
  data: u input; y output
function y = fcn(u)
if(u == 3) %when inverter is in standby state
    y = 0;
elseif(u == 8) %when inverter is in torque control state
    y = 1;
elseif(u==14) %when invertor is in error state
    y = 2;
else
    y = 0;
end

== stateflow chart Clutchless_P2_Parallel_ETE/Clutchless_HSC_ETE/HSC/Powertrain Manager/HV Manager1/DCDC Manager/Chart ==
  state Init
    en:
    DCDC_State = 1;
  state Power_On
    entry: DCmode = 1;
    DCDC_State = 2;
    VoltageHV = 0;
    VoltageLV =14;
    CurrentHV = 20;
    CurrentLV = 173;
  state Delay
    en:
    DCDC_State =2.5;
  state DCDC_Off
    entry: DCDC_State = 3;
    DCmode = 0;
  (default) -> Init
  Init -> Power_On : [ContactorsFailed == 0]
  Delay -> Power_On : after(3,sec)
      | [ContactorsFailed == 0]
  Power_On -> DCDC_Off : [CloseMainC == 0 || INV_state == 14 || ContactorsFailed == 1]
  DCDC_Off -> Delay : [(INV_state == 3 || INV_state == 8)&& (powerMode ==1|| powerMode == 2 || powerMode == 3)]
  data: BMS_IstModus input; CloseMainC input; DCmode output; VoltageHV output; CurrentHV output; VoltageLV output; CurrentLV output; INV_state input; DCDC_State output; EngOnReq input; powerMode input; mode input; keypos input; Contactor local; ContactorsFailed input

== stateflow chart Clutchless_P2_Parallel_ETE/Clutchless_HSC_ETE/HSC/Camaro Fault Detection/Component Diagnostic/Driver Input Diagnostic/Driver_Input_Diag ==
  state Driver_Input_Offline
    en: Driver_Input_Status=0;
  state Driver_Input_Online
    en: Driver_Input_Status=1;
  (default) -> Driver_Input_Offline
  Driver_Input_Online -> Driver_Input_Offline : [~APP_Valid|| ~Drv_BPP_SigValid||~KeyPos||~PRNDL||BrakeFail]
  Driver_Input_Offline -> Driver_Input_Online : [APP_Valid&&Drv_BPP_SigValid&&KeyPos&&PRNDL&&BrakeFail==0]
  data: APP_Valid input; Drv_BPP_SigValid input; KeyPos input; Driver_Input_Status output; PRNDL input; BrakeFail input

== stateflow chart Clutchless_P2_Parallel_ETE/Clutchless_HSC_ETE/HSC/Powertrain Manager/Torque Distribution/EngineCharge Logic ==
  state EngineChg
    entry:
    CDmodeSW=0;
  state Hybrid_Mode
    entry:
    CDmodeSW=1;
  Hybrid_Mode -> EngineChg : [(SW_Engine_On==1&&SW_CS_On ==0)|| (SW_Engine_On == 0 && SW_CS_On == 1)]
  (default) -> Hybrid_Mode
  EngineChg -> Hybrid_Mode : [SW_Engine_On==0 && SW_CS_On==0]
  data: SW_Engine_On input; CDmodeSW output; SW_CS_On input

== stateflow chart Clutchless_P2_Parallel_ETE/Clutchless_HSC_ETE/HSC/Camaro Fault Detection/Component Diagnostic/ESS Component Diagnostic/BMS_CompDiag1 ==
  state BMS_Offline
    en: BMS_Status=0;
  state BMS_Online
    en:BMS_Status=2;
  state BMS_Limited
    en: BMS_Status=1;
  BMS_Offline -> BMS_Online [order 1] : [BMS_RollingAliveActive_SigValid&&BMS_contactorsFailed_SigValid&&...
      | BMS_essTemp_SigValid&&ClearFault&&BMS_essSOC_0_1_SigValid&&...
      | ess_GroundFault&&essCur_A_SigValid]
  (default) -> BMS_Offline
  BMS_Online -> BMS_Offline [order 2] : [~BMS_RollingAliveActive_SigValid||...
      | ~BMS_contactorsFailed_SigValid||~BMS_essSOC_0_1_SigValid|| ...
      | ~ess_GroundFault]
  BMS_Limited -> BMS_Offline [order 2] : [~BMS_RollingAliveActive_SigValid||...
      | ~BMS_contactorsFailed_SigValid]
  BMS_Offline -> BMS_Limited [order 2] : [BMS_RollingAliveActive_SigValid &&...
      | BMS_contactorsFailed_SigValid && ~BMS_essTemp_SigValid||...
      |  ~BMS_essSOC_0_1_SigValid]
  BMS_Limited -> BMS_Online [order 1] : [BMS_essTemp_SigValid||...
      | ClearFault||BMS_essSOC_0_1_SigValid]
  BMS_Online -> BMS_Limited [order 1] : [~BMS_essTemp_SigValid||...
      |  ~BMS_essSOC_0_1_SigValid]
  data: BMS_RollingAliveActive_SigValid input; BMS_contactorsFailed_SigValid input; BMS_essTemp_SigValid input; BMS_Status output; BMS_essSOC_0_1_SigValid input; essCur_A_SigValid input; ess_GroundFault input; ClearFault input

== stateflow chart Clutchless_P2_Parallel_ETE/Clutchless_HSC_ETE/HSC/Camaro Fault Detection/Component Diagnostic/Engine Component Diagnostic/ECM_CompDiag ==
  state ECM_Offline
    en: ECM_Status=0;
  state ECM_Online
    en:ECM_Status=2;
  state ECM_Limited
    en: ECM_Status=1;
  ECM_Online -> ECM_Offline [order 2] : [~ECM_RollingAliveActive||~engTrqCmdRecvd_SigValid||...
      | ~Engine_Speed_rpm_SigValid||Eng_TempRange_123==3||Eng_Torq_Msmch==1||ClearFault==0]
  (default) -> ECM_Offline
  ECM_Offline -> ECM_Online [order 1] : [ECM_RollingAliveActive&&engTrqCmdRecvd_SigValid &&...
      | Engine_Speed_rpm_SigValid&&ClearFault&&Eng_TempRange_123==1&&Eng_Torq_Msmch==0&&ClearFault]
  ECM_Limited -> ECM_Offline [order 2] : [~ECM_RollingAliveActive||~engTrqCmdRecvd_SigValid||~Engine_Speed_rpm_SigValid|| Eng_TempRange_123==3||Eng_Torq_Msmch==1]
  ECM_Offline -> ECM_Limited [order 2] : [ECM_RollingAliveActive...
      | &&engTrqCmdRecvd_SigValid &&Engine_Speed_rpm_SigValid...
      | &&Eng_Torq_Msmch==0&&[Eng_TempRange_123==2 ]]
  ECM_Online -> ECM_Limited [order 1] : [ECM_RollingAliveActive...
      | &&engTrqCmdRecvd_SigValid &&Engine_Speed_rpm_SigValid...
      | &&Eng_Torq_Msmch==0&&(Eng_TempRange_123==2 )]
  ECM_Limited -> ECM_Online [order 1] : [Eng_TempRange_123==1&&Eng_Torq_Msmch==0]
  data: ECM_RollingAliveActive input; engTrqCmdRecvd_SigValid input; Eng_Torq_Msmch input; Engine_Speed_rpm_SigValid input; Eng_TempRange_123 input; ECM_Status output; ClearFault input

== stateflow chart Clutchless_P2_Parallel_ETE/Clutchless_HSC_ETE/HSC/Camaro Fault Detection/Component Diagnostic/Engine Component Diagnostic/Eng_Torq_MsmchLevel ==
  state Normal_Torque
    en: Eng_Torq_MsmchLevel==1
  state Creep_Torq_Allowed
    en: Eng_Torq_MsmchLvel==3
  state AboveMax
    en: Eng_Torq_MsmchLevel==4
  state Max_power_limited
    en: Eng_Torq_MsmchLvel==2
  (default) -> Normal_Torque
  AboveMax -> Normal_Torque [order 2] : [SignalValue<ENGTRQ_MSMCH_Degraded_CP]
  Creep_Torq_Allowed -> AboveMax [order 2] : [SignalValue>ENGTRQ_MSMCH_ErrCritical_CP]
  Max_power_limited -> Normal_Torque [order 1] : [SignalValue<ENGTRQ_MSMCH_Degraded_CP]
  Normal_Torque -> Max_power_limited [order 1] : [SignalValue>ENGTRQ_MSMCH_Degraded_CP&&...
      | SignalValue<ENGTRQ_MSMCH_LimpHome_CP]
  Normal_Torque -> AboveMax [order 2] : [SignalValue>ENGTRQ_MSMCH_ErrCritical_CP]
  AboveMax -> Creep_Torq_Allowed [order 1] : [SignalValue>ENGTRQ_MSMCH_LimpHome_CP&&SignalValue<ENGTRQ_MSMCH_ErrCritical_CP]
  Creep_Torq_Allowed -> Max_power_limited [order 1] : [SignalValue<ENGTRQ_MSMCH_LimpHome_CP&&SignalValue>ENGTRQ_MSMCH_Degraded_CP]
  Max_power_limited -> Creep_Torq_Allowed [order 2] : [SignalValue>ENGTRQ_MSMCH_LimpHome_CP&&SignalValue<ENGTRQ_MSMCH_ErrCritical_CP]
  data: SignalValue input; ENGTRQ_MSMCH_Degraded_CP parameter; ENGTRQ_MSMCH_LimpHome_CP parameter; Eng_Torq_MsmchLevel output; ENGTRQ_MSMCH_ErrCritical_CP parameter

== stateflow chart Clutchless_P2_Parallel_ETE/Clutchless_HSC_ETE/HSC/Camaro Fault Detection/Signal Diagnostic/Driver Signal Diagnostic/AccPedalValidity ==
  state SignalHigh
    en: signalValid=0;
  state SignalInRange
  state SignalLow
    en:signalValid=0;
  SignalHigh -> SignalInRange : [signalValue<=100]
  SignalInRange -> SignalHigh [order 1] : [signalValue>102]
  SignalInRange -> SignalInRange [order 3] : [clearFaults==1]
      | {signalValid=1;}
  (default) -> SignalInRange : {signalValid=1;}
  SignalLow -> SignalInRange : [signalValue>0]
  SignalInRange -> SignalLow [order 2] : [signalValue<-0.5]
  data: clearFaults input; signalValue input; signalValid output

== stateflow chart Clutchless_P2_Parallel_ETE/Clutchless_HSC_ETE/HSC/Powertrain Manager/HV Manager1/BMS_Manager/ESS_Manager ==
  state Ground_Fault
    entry:
    HV_State=-8;
    GFD_Light=1
  state Fault_light_OFF
    entry: GFD_Light=0;
    HV_State=-9;
  state Voltage_Fault
    en:
    HV_State=-11;
  state HVIL_Fault
    entry: MO_BMS_Sollmodus=0;
    HV_State=-10;
  state HV_Startup
    state BMS_Wake
      entry:  HV_State=1;
      T_15=1;
      MO_BMS_Sollmodus=0;
      HVDischarge=0;
    state Clear_Faults
      entry:
      Diag_Rq_Fktnl_Data_OBD_byte_0 =1;
      Diag_Rq_Fktnl_Data_OBD_byte_1=4;
      Diag_Rq_Fktnl_Data_OBD_byte_2=0;
      Diag_Rq_Fktnl_Data_OBD_byte_3=0;
      Diag_Rq_Fktnl_Data_OBD_byte_4=0;
      Diag_Rq_Fktnl_Data_OBD_byte_5=0;
      Diag_Rq_Fktnl_Data_OBD_byte_6=0;
      Diag_Rq_Fktnl_Data_OBD_byte_7=0;
      HV_State=2;
    state Charge_Wake
      entry: chga_wake=1;
      HV_State=3;
    state Drive_Wake
      entry: veh_wake=1;
      HV_State=8;
    state BMS_Enable_Charge
      entry: MO_BMS_Sollmodus=0;
      HV_State=4;
    state BMS_Enable_Drive
      entry: MO_BMS_Sollmodus=0;
      HV_State=9;
    state Power_Contactors_Drive
      en:
      MO_BMS_Sollmodus=0;
      T_30C = 1;
      HV_State=10;
    state Power_Contactors_Charge
      en: MO_BMS_Sollmodus=0;
      T_30C = 1;
      HV_State=5;
    state Close_Contactors_Drive
      entry:
      MO_BMS_Sollmodus=1;
      HV_State=11;
    state Close_Contactors_Charge
      entry:
      MO_BMS_Sollmodus=1;
      HV_State=6;
    state Time_delay
    state Ready_to_Charge
      entry: ReadyToCharge=1;
      ISO_Hybrid_01_Req = 1;
      HV_State=7;
    state Ready_to_Drive
      entry: ReadyToDrive=1;
      ISO_Hybrid_01_Req = 1;
      HV_State=12;
    (default) -> BMS_Wake
    BMS_Wake -> Clear_Faults : after(0.1,sec)
    Clear_Faults -> Charge_Wake [order 1] : [plugged]
    Clear_Faults -> Drive_Wake [order 2] : after(0.15,sec)
    Drive_Wake -> BMS_Enable_Drive : [BMS_Fehler_Pilot==0 ]
    Charge_Wake -> BMS_Enable_Charge : [BMS_Fehler_Pilot==0 ]
    BMS_Enable_Charge -> Power_Contactors_Charge : [BMS_Init_abgeschlossen]
    BMS_Enable_Drive -> Power_Contactors_Drive : [BMS_Init_abgeschlossen]
    Power_Contactors_Drive -> Close_Contactors_Drive : [closeMaincReq]
    Power_Contactors_Charge -> Close_Contactors_Charge : [closeMaincReq]
    Close_Contactors_Charge -> Time_delay : [BMS_Fehler_HS_offen==0&&(BMS_IstModus==4||BMS_IstModus==1)]
    Close_Contactors_Drive -> Ready_to_Drive : [BMS_Fehler_HS_offen==0&&BMS_IstModus==1]
    Time_delay -> Ready_to_Charge : after(1,sec)
    Ready_to_Drive -> Ready_to_Charge : [plugged]
    Ready_to_Charge -> Ready_to_Drive : [plugged==0]
  note: // Rev 2_14_2017
      | Added plugged to Off-On transition
      | Added EnableInverter to charge path
      | Changed IstModus to 1 at the end of charge path
      |
      | Create HV On Request block to request charging when vehicle is off
  state HV_Shudown
    state MCU_Delay
      en:
      HV_State = -1;
    state Open_Contactors
      entry: MO_BMS_Sollmodus=0;
      HV_State=-2;
      ISO_Hybrid_01_Req = 0;
    state ShutDown_T30C
      entry: T_30C=0;
    state Discharge_Bus
      entry: HVDischarge=1;
      HV_State=-3;
    state Disable_BCM_1
      entry: T_15=0;
      HVDischarge=0;
      HV_State=-4;
    state Disable_BCM_2
      entry: T_30=0;
      HVDischarge=0;
      HV_State=-5;
    state Send_BCM_to_Sleep
      en: MO_SleepAckn =1;
      T_15=0;
      T_30=0;
      HV_State=-6;
    state Shutdown_Complete
      entry: Shutdown_Complete=1;
      HV_State=-7;
    (default) -> MCU_Delay
    MCU_Delay -> Open_Contactors : [MCU_State >= 9]
    Open_Contactors -> ShutDown_T30C : after(2,sec)
    ShutDown_T30C -> Discharge_Bus : [BMS_IstModus==5]
    Discharge_Bus -> Disable_BCM_1 : [BMS_Spannung_ZwKr<30]
    Disable_BCM_1 -> Disable_BCM_2 : [BMS_IstStrom<0.02]
    Disable_BCM_2 -> Send_BCM_to_Sleep
    Send_BCM_to_Sleep -> Shutdown_Complete : [BMS_SleepInd]
  note: //Rev 8_21_2017
      | //Removed all engine related conditions
      | //Removed EngRunATV
  Voltage_Fault -> HV_Shudown : after(0.25, sec)
  Ground_Fault -> Fault_light_OFF : [(ISOfault==0&&KeyPos==1)||(ISOfault==0&&KeyPos==0&&plugged==1)]
  HV_Shudown -> Ground_Fault [order 2] : [ISOfault==1]
  Fault_light_OFF -> HV_Shudown
  HV_Startup -> Ground_Fault [order 3] : [ISOfault==1]
  HV_Startup -> HVIL_Fault [order 4] : [BMS_Fehler_Pilot]
  HVIL_Fault -> HV_Shudown : [BMS_Fehler_Pilot==0]
  HV_Startup -> Voltage_Fault [order 1] : after(5,sec)
      | [BMS_Spannung_ZwKr<50&&EngRunAtv]
  (default) -> HV_Shudown
  HV_Shudown -> HV_Startup [order 1] : [HV_req==1||plugged||EngRunAtv]
  HV_Startup -> HV_Shudown [order 2] : [(HV_req==0 && plugged==0) || SoC < 10]
      | {ReadyToDrive = 0;
      | ReadyToCharge = 0;}
  data: data local; ISOfault input; plugged input; BMS_Fehler_HS_offen input; BMS_Fehler_Pilot input; BMS_Init_abgeschlossen input; BMS_IstModus input; BMS_IstSpannung input; BMS_IstStrom input; BMS_SleepInd input; Diag_Rq_Fktnl_Data_OBD_byte_0 output; Diag_Rq_Fktnl_Data_OBD_byte_1 output; Diag_Rq_Fktnl_Data_OBD_byte_2 output; Diag_Rq_Fktnl_Data_OBD_byte_3 output; Diag_Rq_Fktnl_Data_OBD_byte_4 output; Diag_Rq_Fktnl_Data_OBD_byte_5 output; Diag_Rq_Fktnl_Data_OBD_byte_6 output; Diag_Rq_Fktnl_Data_OBD_byte_7 output; ISO_Hybrid_01_Req output; MO_SleepAckn output; MO_BMS_Sollmodus output; T_15 output; T_30 output; T_30C output; veh_wake output; chga_wake output; HVDischarge output; HV_State output; ReadyToDrive output; ReadyToCharge output; Shutdown_Complete output; HV_req input boolean; BMS_Spannung_ZwKr input; NMH_BMS_Car_WakeUp input; NMH_Normal_Mode_1 input; NMH_BMS_Normal_Mode_2 input; NMH_BMS_Start_1 input; NMH_BMS_Start_2 input; timer local; KeyPos input; GFD_Light output; EngRunAtv input; closeMaincReq input boolean; INV_State input; SoC input; MCU_State input

== stateflow chart Clutchless_P2_Parallel_ETE/Clutchless_HSC_ETE/HSC/Camaro Fault Detection/Signal Diagnostic/Driver Signal Diagnostic/AccPedalValidity1 ==
  state SignalHigh
    en: signalValid=0;
  state SignalInRange
  state SignalLow
    en:signalValid=0;
  SignalHigh -> SignalInRange : [signalValue<=100]
  SignalInRange -> SignalHigh [order 1] : [signalValue>102]
  SignalInRange -> SignalInRange [order 3] : [clearFaults==1]
      | {signalValid=1;}
  (default) -> SignalInRange : {signalValid=1;}
  SignalLow -> SignalInRange : [signalValue>0]
  SignalInRange -> SignalLow [order 2] : [signalValue<-0.5]
  data: clearFaults input; signalValue input; signalValid output

== stateflow chart Clutchless_P2_Parallel_ETE/Clutchless_HSC_ETE/HSC/Camaro Fault Detection/Signal Diagnostic/Driver Signal Diagnostic/BrakeFailureDetection/Chart ==
  state No_Fault
    en:
    DecelFail=0;
  state Detection_State
    en:
    Detection_state=1;
  state No_Fault1
    en:
    DecelFail=0;
  state Detection_State1
    en:
    Detection_state=2;
  state No_Fault2
    en:
    DecelFail=0;
  state Detection_State2
    en:
    Detection_state=3;
    du:
    DecelFail=1;
  (default) -> (junction 3)
  (junction 3) -> No_Fault [order 2]
  (junction 3) -> Detection_State [order 1] : [VehSpeed>0]
  Detection_State -> (junction 8)
  (junction 8) -> No_Fault1 [order 2]
  (junction 8) -> Detection_State1 [order 1] : [BPP>0]
  Detection_State1 -> (junction 15)
  (junction 15) -> No_Fault2 [order 2]
  (junction 15) -> Detection_State2 [order 1] : [Incre||Unchange]
  data: BPP input; VehSpeed input; Incre input; Unchange input; DecelFail output; Detection_state local
